simulink model "simulink_q3"  (R2024b)
settings: Solver=VariableStepAuto  StartTime=0.0  StopTime=10  RelTol=1e-3
values from neighbouring files (symbols this model uses):
  U0 = [0.525841853692 -0.00469375602825 0 0 0]    [ICs_aircraft2_180Kts_CG1.mat]    (also in ICs_aircraft2_180Kts_CG2.mat = [0.525939752377 -0.00596702425354 0 0 0]; ICs_aircraft2_75Kts_CG1.mat = [0.0938327586982 -0.025121721174 0 0 0]; ICs_aircraft2_75Kts_CG2.mat = [0.0933937108451 -0.0325384431522 0 0 0])
undefined symbols (not defined in the file or in its folder): FlightData
libraries: cstblocks x3, slpidlib x1
settings Model: Creator=ben83  LastModifiedBy=Bez
settings RTWCC: GPUComputeCapability=3.5

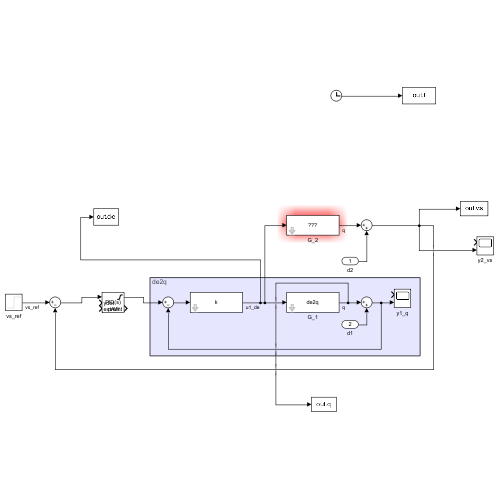
[thumbnail: Simulink's stored preview of the top-level diagram]
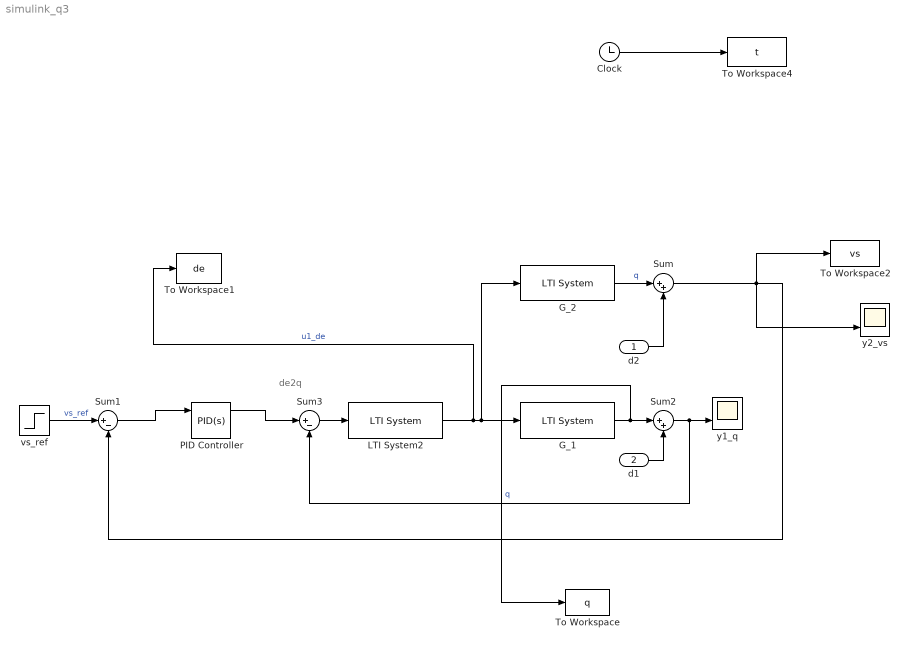
== system simulink_q3 ==
  note: de2q
  d2 : Inport
  d1 : Inport  Port=2
  Clock : Clock
  G_1 : cstblocks/LTI System  sys=de2q  IC=[]  PadeOrder=0
  G_2 : cstblocks/LTI System  sys=de2vs  IC=[]  PadeOrder=0
  LTI System2 : cstblocks/LTI System  sys=k  IC=[]  PadeOrder=0
  PID Controller : slpidlib/PID Controller  Controller=PID  Form=Parallel  TimeDomain=Continuous-time  UseExternalTs=off  SampleTime=-1  IntegratorMethod=Forward Euler  FilterMethod=Forward Euler  ControllerParametersSource=internal  P=0.0551848259607478  I=0.0116620584429928  UseKiTs=off  D=0.0284828891496478  UseExternalDerivativeSource=on  N=228.565595208321  UseFilter=on  TunerSelectOption=Transfer Function Based (PID Tuner App)  InitialConditionSource=internal  InitialConditionForIntegrator=0  InitialConditionForFilter=0  DifferentiatorICPrevScaledInput=0  ExternalReset=none  TrackingMode=off  Kt=1  LimitOutput=on  SatLimitsSource=internal  UpperSaturationLimit=FlightData.CntrlLimit.Upper(2,:)  LowerSaturationLimit=FlightData.CntrlLimit.Lower(2,:)  LinearizeAsGain=on  AntiWindupMode=external  Kb=1  LimitIntegrator=off  UpperIntegratorSaturationLimit=inf  LowerIntegratorSaturationLimit=-inf  POutMin=[]  POutMax=[]  IOutMin=[]  IOutMax=[]  DOutMin=[]  DOutMax=[]  NOutMin=[]  NOutMax=[]  SumOutMin=[]  SumOutMax=[]  SaturationOutMin=[]  SaturationOutMax=[]  PParamMin=[]  PParamMax=[]  IParamMin=[]  IParamMax=[]  DParamMin=[]  DParamMax=[]  NParamMin=[]  NParamMax=[]  KbParamMin=[]  KbParamMax=[]  KtParamMin=[]  KtParamMax=[]  KbOutMin=[]  KbOutMax=[]  KtOutMin=[]  KtOutMax=[]  IntegratorOutMin=[]  IntegratorOutMax=[]  FilterOutMin=[]  FilterOutMax=[]  SumI1OutMin=[]  SumI1OutMax=[]  SumI2OutMin=[]  SumI2OutMax=[]  SumI3OutMin=[]  SumI3OutMax=[]  SumI4OutMin=[]  SumI4OutMax=[]  SumDOutMin=[]  SumDOutMax=[]  DifferentiatorOutMin=[]  DifferentiatorOutMax=[]  FilterDiffOutCoefMin=[]  FilterDiffOutCoefMax=[]  ReciprocalOutMin=[]  ReciprocalOutMax=[]  SumDenOutMin=[]  SumDenOutMax=[]  SumNumOutMin=[]  SumNumOutMax=[]  DivideOutMin=[]  DivideOutMax=[]  UdiffTsProdOutMin=[]  UdiffTsProdOutMax=[]  NTsProdOutMin=[]  NTsProdOutMax=[]  UintegralTsProdOutMin=[]  UintegralTsProdOutMax=[]  UngainTsProdOutMin=[]  UngainTsProdOutMax=[]  ClampingZeroOutDataTypeStr=Inherit: Inherit via back propagation  ClampingZeroOutMin=[]  ClampingZeroOutMax=[]  FilterDenConstantOutDataTypeStr=Inherit: Inherit via back propagation  FilterDenConstantOutMin=[]  FilterDenConstantOutMax=[]  PCopyOutDataTypeStr=Inherit: Inherit via back propagation  PCopyOutMin=[]  PCopyOutMax=[]  NCopyOutDataTypeStr=Inherit: Inherit via back propagation  NCopyOutMin=[]  NCopyOutMax=[]  IntegratorContinuousStateAttributes=''  IntegratorStateMustResolveToSignalObject=off  IntegratorRTWStateStorageClass=Auto  FilterContinuousStateAttributes=''  FilterStateMustResolveToSignalObject=off  FilterRTWStateStorageClass=Auto  ParallelPVariant=InternalParameters  IdealPVariant=Disabled  IVariant=InternalParameters  DVariant=InternalParameters  IntegratorVariant=Continuous  SatVariant=Disabled  AWVariant=Passthrough  PCopyVariant=Disabled  TRVariant=Disabled  FdbkBlocksVariant=Forward  IdealPFdbkVariant=Disabled  SatFdbkVariant=Disabled  DerivativeFilterVariant=ContFilter  NVariant=InternalParameters  NCopyVariant=Disabled  FilterICVariant=InternalICsFilter  IntegratorICVariant=InternalICs  ExternalResetVariant=Disabled  TRSumVariant=Passthrough  SumFdbkVariant=Disabled  SumVariant=Sum_PID  TsampFilterVariant=InternalTs  TsampNgainVariant=Passthrough  TsampIntegralVariant=Passthrough  ExternalSaturationOutDataTypeStr=Inherit: Same as second input  DerivativeSourceVariant=ErrorSignal  PreIntVariant=InternalPreInt
  Sum : Sum  Inputs=|++
  Sum1 : Sum  Inputs=|+-
  Sum2 : Sum  Inputs=|++
  Sum3 : Sum  Inputs=|+-
  To Workspace : ToWorkspace  VariableName=q  SampleTime=-1
  To Workspace1 : ToWorkspace  VariableName=de  SampleTime=-1
  To Workspace2 : ToWorkspace  VariableName=vs  SampleTime=-1
  To Workspace4 : ToWorkspace  VariableName=t  SampleTime=-1
  vs_ref : Step  Before=U0(2,:)  After=8.3  SampleTime=0.01
  y1_q : Scope  NumInputPorts=2
  y2_vs : Scope  NumInputPorts=2
  wires:
  Sum3/1 -> LTI System2/1
  LTI System2/1 -> To Workspace1/1, G_2/1, G_1/1  "u1_de"
  vs_ref/1 -> Sum1/1  "vs_ref"
  G_2/1 -> Sum/1  "q"
  d1/1 -> Sum2/2
  d2/1 -> Sum/2
  Sum2/1 -> Sum3/2, y1_q/2
  G_1/1 -> To Workspace/1, Sum2/1  "q"
  Sum/1 -> To Workspace2/1, y2_vs/2, Sum1/2
  Sum1/1 -> PID Controller/1
  PID Controller/1 -> Sum3/1
  Clock/1 -> To Workspace4/1
